simulink model "mvdc_KF_PointMassJoint"  (R2018b)
settings: configuration reference "Active" (kept outside this file)
undefined symbols (not defined in the file): P_VDC_EnableInputCrossCorrelation, P_VDC_InputCov, P_VDC_ManualInitializationStartPose, P_VDC_ManualInitializationStateEstimation, P_VDC_MeasCov, P_VDC_OutlierBounds, P_VDC_ResFilterSamples, P_VDC_resLim_psiLoc1_rad, P_VDC_resLim_psiLoc2_rad, P_VDC_resLim_vxVel1_mps, P_VDC_resLim_vxVel2_mps, P_VDC_resLim_vyVel1_mps, P_VDC_resLim_vyVel2_mps, P_VDC_resLim_xLoc1_m, P_VDC_resLim_xLoc2_m, P_VDC_resLim_yLoc1_m, P_VDC_resLim_yLoc2_m, P_VDC_YawAngleDepCovMode, res_dLoc1_m, res_dLoc2_m, res_dPsi1_radps, res_dPsi2_radps, res_psiLoc1_rad, res_psiLoc2_rad, res_sLoc1_m, res_sLoc2_m, res_vxVel1_mps, res_vxVel2_mps, res_vyVel1_mps, res_vyVel2_mps, res_xLoc1_m, res_xLoc2_m, res_yLoc1_m, res_yLoc2_m, tS
libraries: simulink x12
settings Model: DataDictionary=mvdc_KF_PointMassJoint.sldd  Creator=Madeline  LastModifiedBy=ge34qer

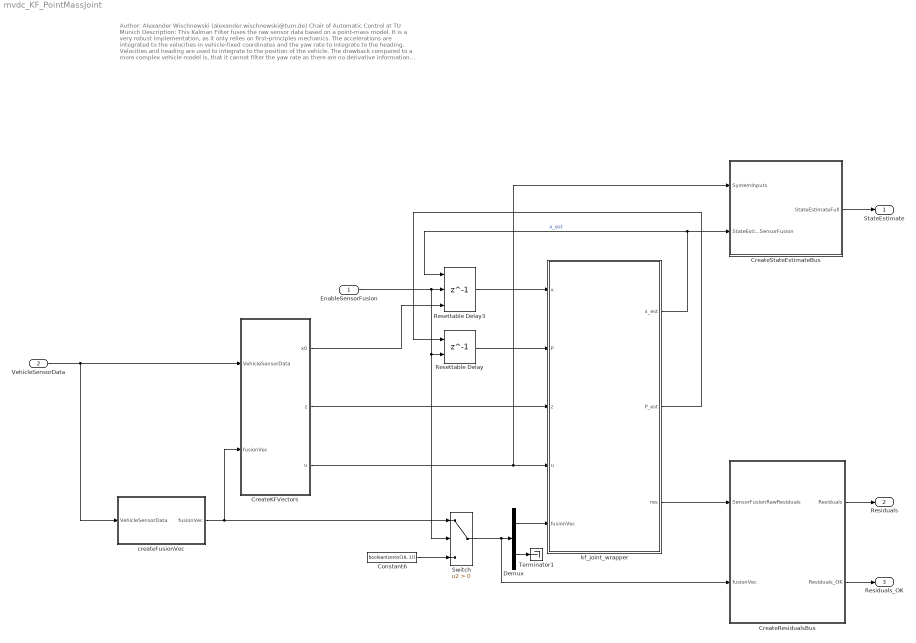
== system mvdc_KF_PointMassJoint ==
  note: Author: Alexander Wischnewski (alexander.wischnewski@tum.de)
      | Chair of Automatic Control at TU Munich
      |
      | Description: This Kalman Filter fuses the raw sensor data based on a point-mass model. It is a very robust implementation, as it only relies on first-principles mechanics. The accelerations are integrated to the velocities in vehicle-fixed coordinates and the yaw rate to integrate to the heading. Velocities and heading are used to integrate to the position of the vehicle. The drawback compared to a more complex vehicle model is, that it cannot filter the yaw rate as there are no derivative information about the yaw rate available. However, it is easy to tune and has comparable performance over the whole range of operating points.
      |
      | Inputs:
      | EnableSensorFusion Enable bit which activates the Kalman Filter
      | VehicleSensorData Raw sensor data
      |
      | Outputs:
      | StateEstimate Estimated state vector of the Kalman Filter
      | Residuals Pre-update measurement residuals of the Kalman Filter
      | Covariances Post-update Estimation Covariance Matrix of the Kalman Filter
  EnableSensorFusion : Inport  OutDataTypeStr=boolean
  VehicleSensorData : Inport  Port=2  OutDataTypeStr=Bus: VehicleSensorData
  Constant6 : Constant  Value=boolean(zeros(16, 1))
  CreateKFVectors : Subsystem
  CreateResidualsBus : Subsystem
  CreateStateEstimateBus : Subsystem
  Demux : Demux  Outputs=[10 6]
  Resettable Delay : Delay  DelayLength=1  InitialCondition=eye(5)*0.1  ExternalReset=Rising
      settings: InputPortMap=u0,r5
  Resettable Delay3 : Delay  DelayLength=1  InitialConditionSource=Input port  ExternalReset=Rising
      settings: InputPortMap=u0,r5,p4
  Switch : Switch  Criteria=u2 > Threshold
  Terminator1 : Terminator
  createFusionVec : Subsystem
  kf_joint_wrapper : MATLAB Function  TreatAsAtomicUnit=on
  "StateEstimate " : Outport  OutDataTypeStr=Bus: StateEstimation_state
  Residuals : Outport  Port=2  OutDataTypeStr=Bus: StateEstimation_residuals
  Residuals_OK : Outport  Port=3  OutDataTypeStr=boolean
  wires:
  kf_joint_wrapper/1(x_est) -> Resettable Delay3/1, CreateStateEstimateBus/2(StateEstimateSensorFusion)  "x_est"
  Resettable Delay3/1 -> kf_joint_wrapper/1(x)
  kf_joint_wrapper/2(P_est) -> Resettable Delay/1
  Resettable Delay/1 -> kf_joint_wrapper/2(P)
  CreateResidualsBus/1(Residuals) -> Residuals/1
  CreateKFVectors/1(x0) -> Resettable Delay3/3
  VehicleSensorData/1 -> createFusionVec/1(VehicleSensorData), CreateKFVectors/1(VehicleSensorData)
  CreateKFVectors/2(z) -> kf_joint_wrapper/3(z)
  CreateKFVectors/3(u) -> CreateStateEstimateBus/1(SystemInputs), kf_joint_wrapper/4(u)
  CreateStateEstimateBus/1(StateEstimateFull) -> "StateEstimate "/1
  kf_joint_wrapper/3(res) -> CreateResidualsBus/1(SensorFusionRawResiduals)
  Demux/2 -> Terminator1/1
  Demux/1 -> kf_joint_wrapper/5(fusionVec)
  Constant6/1 -> Switch/3
  EnableSensorFusion/1 -> Switch/2, Resettable Delay/2, Resettable Delay3/2
  createFusionVec/1(fusionVec) -> CreateKFVectors/2(fusionVec), Switch/1
  Switch/1 -> CreateResidualsBus/2(fusionVec), Demux/1
  CreateResidualsBus/2(Residuals_OK) -> Residuals_OK/1

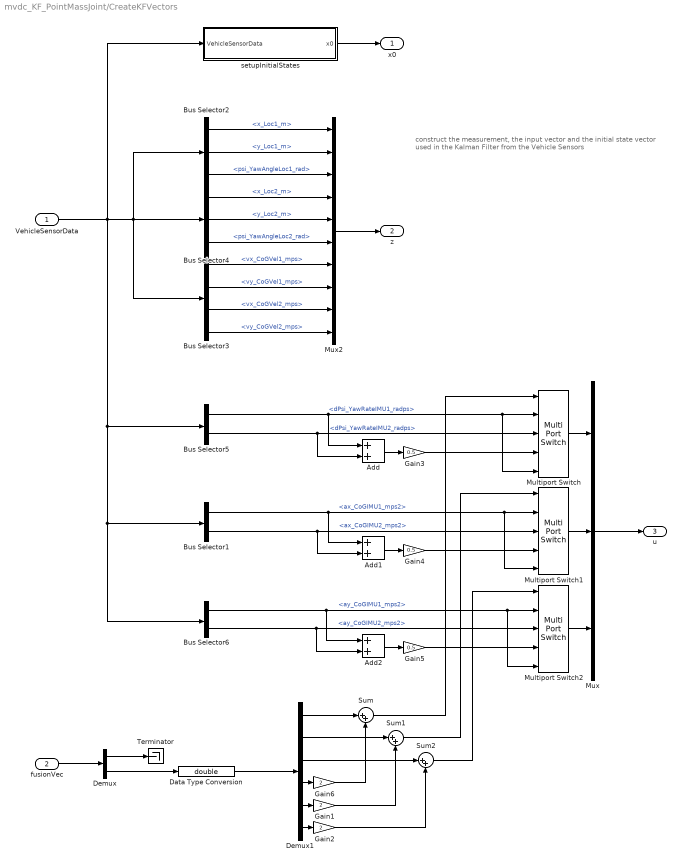
== system mvdc_KF_PointMassJoint/CreateKFVectors ==
  note: construct the measurement, the input vector and the initial state vector
      | used in the Kalman Filter from the Vehicle Sensors
  VehicleSensorData : Inport
  fusionVec : Inport  Port=2  OutDataTypeStr=boolean  PortDimensions=16
  Add : Sum
  Add1 : Sum
  Add2 : Sum
  Bus Selector1 : BusSelector  OutputSignals=ax_CoGIMU1_mps2,ax_CoGIMU2_mps2
  Bus Selector2 : BusSelector  OutputSignals=x_Loc1_m,y_Loc1_m,psi_YawAngleLoc1_rad
  Bus Selector3 : BusSelector  OutputSignals=vx_CoGVel1_mps,vy_CoGVel1_mps,vx_CoGVel2_mps,vy_CoGVel2_mps
  Bus Selector4 : BusSelector  OutputSignals=x_Loc2_m,y_Loc2_m,psi_YawAngleLoc2_rad
  Bus Selector5 : BusSelector  OutputSignals=dPsi_YawRateIMU1_radps,dPsi_YawRateIMU2_radps
  Bus Selector6 : BusSelector  OutputSignals=ay_CoGIMU1_mps2,ay_CoGIMU2_mps2
  Data Type Conversion : DataTypeConversion  OutDataTypeStr=double
  Demux : Demux  Outputs=[10 6]
  Demux1 : Demux  Outputs=6
  Gain1 : Gain  Gain=2
  Gain2 : Gain  Gain=2
  Gain3 : Gain  Gain=0.5
  Gain4 : Gain  Gain=0.5
  Gain5 : Gain  Gain=0.5
  Gain6 : Gain  Gain=2
  Multiport Switch : MultiPortSwitch  DataPortForDefault=Additional data port  DiagnosticForDefault=Warning
  Multiport Switch1 : MultiPortSwitch  DataPortForDefault=Additional data port  DiagnosticForDefault=Warning
  Multiport Switch2 : MultiPortSwitch  DataPortForDefault=Additional data port  DiagnosticForDefault=Warning
  Mux : Mux  Inputs=3
  Mux2 : Mux  Inputs=10
  Sum : Sum  Inputs=|++
  Sum1 : Sum  Inputs=|++
  Sum2 : Sum  Inputs=|++
  Terminator : Terminator
  setupInitialStates : Subsystem
  x0 : Outport
  z : Outport  Port=2
  u : Outport  Port=3
  wires:
  Mux2/1 -> z/1
  Bus Selector4/1 -> Mux2/4  "<x_Loc2_m>"
  Bus Selector4/2 -> Mux2/5  "<y_Loc2_m>"
  Bus Selector2/3 -> Mux2/3  "<psi_YawAngleLoc1_rad>"
  Bus Selector4/3 -> Mux2/6  "<psi_YawAngleLoc2_rad>"
  Bus Selector2/2 -> Mux2/2  "<y_Loc1_m>"
  Bus Selector2/1 -> Mux2/1  "<x_Loc1_m>"
  Bus Selector3/1 -> Mux2/7  "<vx_CoGVel1_mps>"
  Bus Selector3/2 -> Mux2/8  "<vy_CoGVel1_mps>"
  Bus Selector3/3 -> Mux2/9  "<vx_CoGVel2_mps>"
  Bus Selector3/4 -> Mux2/10  "<vy_CoGVel2_mps>"
  setupInitialStates/1(x0) -> x0/1
  Mux/1 -> u/1
  Demux/1 -> Terminator/1
  Demux/2 -> Data Type Conversion/1
  Demux1/6 -> Gain2/1
  Demux1/1 -> Sum/1
  Demux1/2 -> Sum1/1
  Demux1/3 -> Sum2/1
  Bus Selector5/1 -> Add/1, Multiport Switch/5, Multiport Switch/2  "<dPsi_YawRateIMU1_radps>"
  Bus Selector5/2 -> Add/2, Multiport Switch/3  "<dPsi_YawRateIMU2_radps>"
  Add/1 -> Gain3/1
  Sum/1 -> Multiport Switch/1
  Multiport Switch/1 -> Mux/1
  Multiport Switch1/1 -> Mux/2
  VehicleSensorData/1 -> setupInitialStates/1(VehicleSensorData), Bus Selector6/1, Bus Selector1/1, Bus Selector5/1, Bus Selector2/1, Bus Selector3/1, Bus Selector4/1
  Sum1/1 -> Multiport Switch1/1
  Bus Selector6/1 -> Add2/1, Multiport Switch2/5, Multiport Switch2/2  "<ay_CoGIMU1_mps2>"
  Add2/1 -> Gain5/1
  Gain5/1 -> Multiport Switch2/4
  Bus Selector6/2 -> Add2/2, Multiport Switch2/3  "<ay_CoGIMU2_mps2>"
  Multiport Switch2/1 -> Mux/3
  Sum2/1 -> Multiport Switch2/1
  Demux1/5 -> Gain1/1
  Demux1/4 -> Gain6/1
  Gain6/1 -> Sum/2
  Gain1/1 -> Sum1/2
  Gain2/1 -> Sum2/2
  Gain3/1 -> Multiport Switch/4
  Bus Selector1/2 -> Add1/2, Multiport Switch1/3  "<ax_CoGIMU2_mps2>"
  Add1/1 -> Gain4/1
  Bus Selector1/1 -> Add1/1, Multiport Switch1/5, Multiport Switch1/2  "<ax_CoGIMU1_mps2>"
  Gain4/1 -> Multiport Switch1/4
  Data Type Conversion/1 -> Demux1/1
  fusionVec/1 -> Demux/1

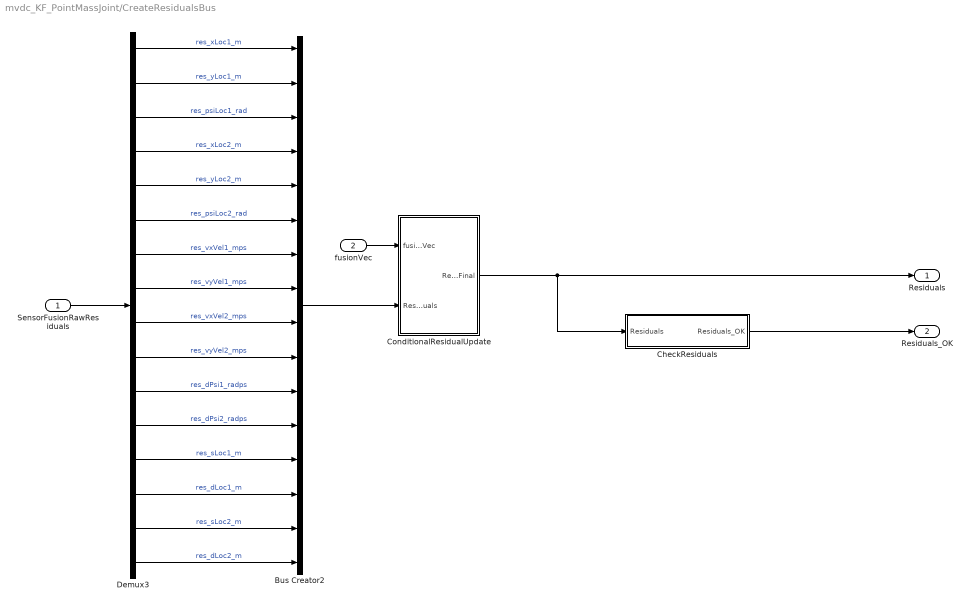
== system mvdc_KF_PointMassJoint/CreateResidualsBus ==
  SensorFusionRawResiduals : Inport
  fusionVec : Inport  Port=2
  Bus Creator2 : BusCreator  Inputs=16
  CheckResiduals : Subsystem
  ConditionalResidualUpdate : Subsystem
  Demux3 : Demux  Outputs=16
  Residuals : Outport
  Residuals_OK : Outport  Port=2  OutDataTypeStr=boolean
  wires:
  Demux3/3 -> Bus Creator2/3  "res_psiLoc1_rad"
  Demux3/1 -> Bus Creator2/1  "res_xLoc1_m"
  Demux3/2 -> Bus Creator2/2  "res_yLoc1_m"
  Demux3/13 -> Bus Creator2/13  "res_sLoc1_m"
  Demux3/14 -> Bus Creator2/14  "res_dLoc1_m"
  Demux3/15 -> Bus Creator2/15  "res_sLoc2_m"
  Demux3/16 -> Bus Creator2/16  "res_dLoc2_m"
  fusionVec/1 -> ConditionalResidualUpdate/1(fusionVec)
  SensorFusionRawResiduals/1 -> Demux3/1
  Bus Creator2/1 -> ConditionalResidualUpdate/2(Residuals)
  Demux3/4 -> Bus Creator2/4  "res_xLoc2_m"
  Demux3/5 -> Bus Creator2/5  "res_yLoc2_m"
  Demux3/6 -> Bus Creator2/6  "res_psiLoc2_rad"
  Demux3/7 -> Bus Creator2/7  "res_vxVel1_mps"
  Demux3/8 -> Bus Creator2/8  "res_vyVel1_mps"
  Demux3/11 -> Bus Creator2/11  "res_dPsi1_radps"
  Demux3/9 -> Bus Creator2/9  "res_vxVel2_mps"
  Demux3/10 -> Bus Creator2/10  "res_vyVel2_mps"
  Demux3/12 -> Bus Creator2/12  "res_dPsi2_radps"
  ConditionalResidualUpdate/1(ResidualsFinal) -> CheckResiduals/1(Residuals), Residuals/1
  CheckResiduals/1(Residuals_OK) -> Residuals_OK/1

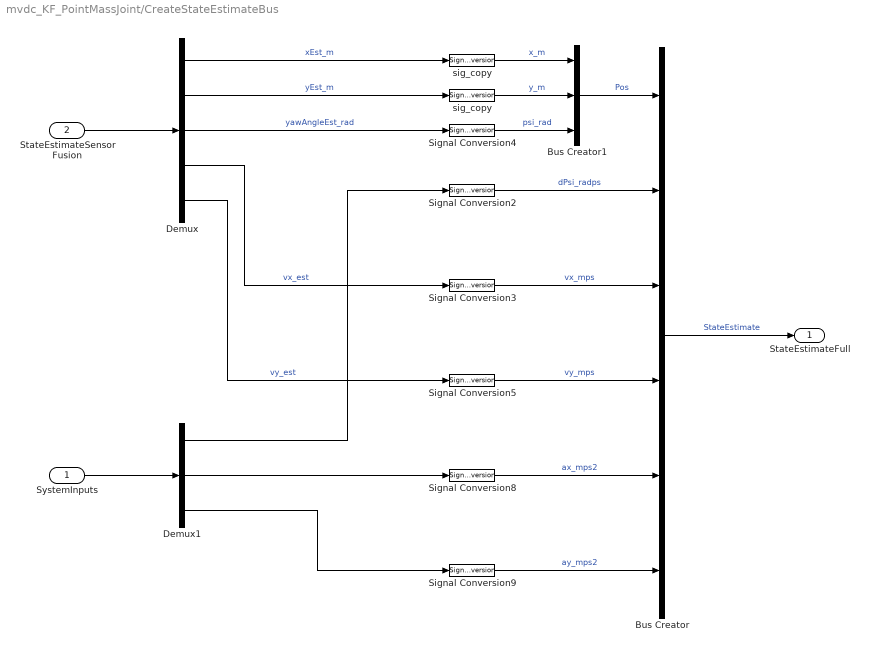
== system mvdc_KF_PointMassJoint/CreateStateEstimateBus ==
  SystemInputs : Inport
  StateEstimateSensorFusion : Inport  Port=2
  Bus Creator : BusCreator  Inputs=6
  Bus Creator1 : BusCreator  Inputs=3  OutDataTypeStr=Bus: CartPos
  Demux : Demux  Outputs=5
  Demux1 : Demux  Outputs=3
  Signal Conversion{2..5,8..9} (6 alike) : SignalConversion  OverrideOpt=off
  sig_copy : SignalConversion  OverrideOpt=off
  "sig_copy " : SignalConversion  OverrideOpt=off
  StateEstimateFull : Outport
  wires:
  StateEstimateSensorFusion/1 -> Demux/1
  Demux/1 -> "sig_copy "/1  "xEst_m"
  "sig_copy "/1 -> Bus Creator1/1  "x_m"
  Demux/3 -> Signal Conversion4/1  "yawAngleEst_rad"
  Demux/2 -> sig_copy/1  "yEst_m"
  Bus Creator/1 -> StateEstimateFull/1  "StateEstimate"
  Bus Creator1/1 -> Bus Creator/1  "Pos"
  Signal Conversion4/1 -> Bus Creator1/3  "psi_rad"
  Signal Conversion3/1 -> Bus Creator/3  "vx_mps"
  Signal Conversion2/1 -> Bus Creator/2  "dPsi_radps"
  Signal Conversion8/1 -> Bus Creator/5  "ax_mps2"
  Signal Conversion9/1 -> Bus Creator/6  "ay_mps2"
  Signal Conversion5/1 -> Bus Creator/4  "vy_mps"
  sig_copy/1 -> Bus Creator1/2  "y_m"
  Demux/5 -> Signal Conversion5/1  "vy_est"
  Demux/4 -> Signal Conversion3/1  "vx_est"
  SystemInputs/1 -> Demux1/1
  Demux1/1 -> Signal Conversion2/1
  Demux1/2 -> Signal Conversion8/1
  Demux1/3 -> Signal Conversion9/1

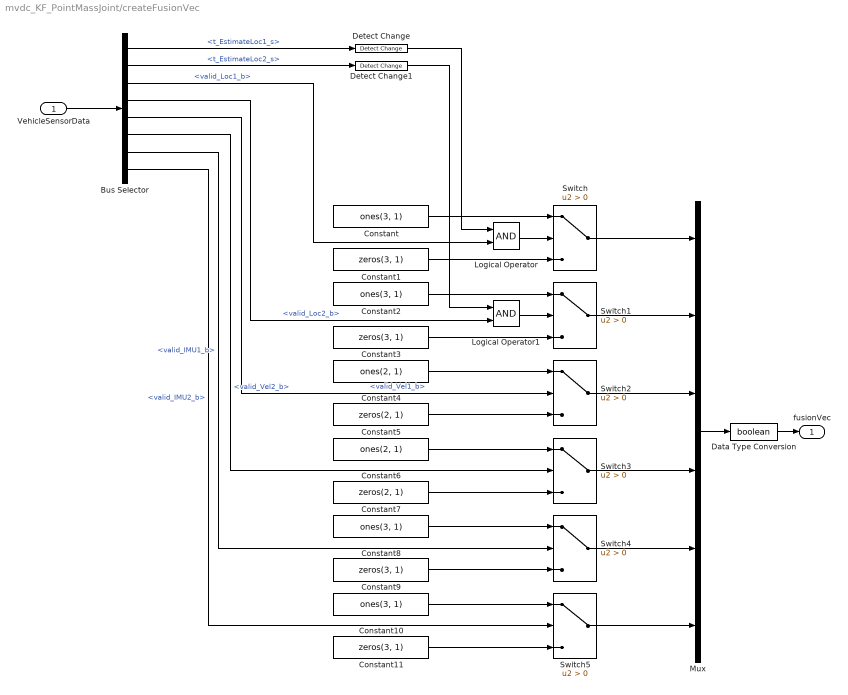
== system mvdc_KF_PointMassJoint/createFusionVec ==
  VehicleSensorData : Inport
  Bus Selector : BusSelector  OutputSignals=t_EstimateLoc1_s,t_EstimateLoc2_s,valid_Loc1_b,valid_Loc2_b,valid_Vel1_b,valid_Vel2_b,valid_IMU1_b,valid_IMU2_b
  Constant{,2,8,10} (4 alike) : Constant  Value=ones(3, 1)
  Constant{1,3,9,11} (4 alike) : Constant  Value=zeros(3, 1)
  Constant4 : Constant  Value=ones(2, 1)
  Constant5 : Constant  Value=zeros(2, 1)
  Constant6 : Constant  Value=ones(2, 1)
  Constant7 : Constant  Value=zeros(2, 1)
  Data Type Conversion : DataTypeConversion  OutDataTypeStr=boolean
  Detect Change : simulink/Logic and Bit Operations/Detect Change  vinit=0  OutDataTypeStr=boolean
  Detect Change1 : simulink/Logic and Bit Operations/Detect Change  vinit=0  OutDataTypeStr=boolean
  Logical Operator : Logic  AllPortsSameDT=off  OutDataTypeStr=boolean
  Logical Operator1 : Logic  AllPortsSameDT=off  OutDataTypeStr=boolean
  Mux : Mux  Inputs=6
  Switch{,1..5} (6 alike) : Switch  Criteria=u2 > Threshold
  fusionVec : Outport
  wires:
  Switch5/1 -> Mux/6
  Constant7/1 -> Switch3/3
  Switch2/1 -> Mux/3
  Constant8/1 -> Switch4/1
  Constant6/1 -> Switch3/1
  Constant1/1 -> Switch/3
  Constant2/1 -> Switch1/1
  Constant11/1 -> Switch5/3
  Switch3/1 -> Mux/4
  Switch4/1 -> Mux/5
  Constant9/1 -> Switch4/3
  Constant5/1 -> Switch2/3
  Constant/1 -> Switch/1
  Constant10/1 -> Switch5/1
  Switch/1 -> Mux/1
  Constant4/1 -> Switch2/1
  Switch1/1 -> Mux/2
  Constant3/1 -> Switch1/3
  Data Type Conversion/1 -> fusionVec/1
  Mux/1 -> Data Type Conversion/1
  Logical Operator/1 -> Switch/2
  Logical Operator1/1 -> Switch1/2
  VehicleSensorData/1 -> Bus Selector/1
  Bus Selector/1 -> Detect Change/1  "<t_EstimateLoc1_s>"
  Bus Selector/2 -> Detect Change1/1  "<t_EstimateLoc2_s>"
  Detect Change/1 -> Logical Operator/1
  Detect Change1/1 -> Logical Operator1/1
  Bus Selector/3 -> Logical Operator/2  "<valid_Loc1_b>"
  Bus Selector/4 -> Logical Operator1/2  "<valid_Loc2_b>"
  Bus Selector/5 -> Switch2/2  "<valid_Vel1_b>"
  Bus Selector/6 -> Switch3/2  "<valid_Vel2_b>"
  Bus Selector/7 -> Switch4/2  "<valid_IMU1_b>"
  Bus Selector/8 -> Switch5/2  "<valid_IMU2_b>"

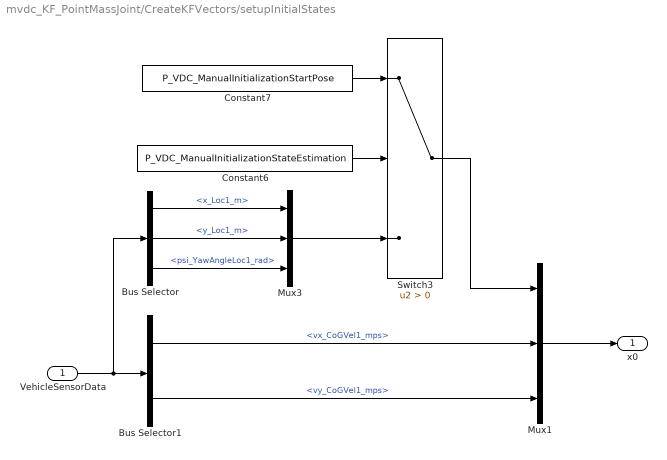
== system mvdc_KF_PointMassJoint/CreateKFVectors/setupInitialStates ==
  VehicleSensorData : Inport
  Bus Selector : BusSelector  OutputSignals=x_Loc1_m,y_Loc1_m,psi_YawAngleLoc1_rad
  Bus Selector1 : BusSelector  OutputSignals=vx_CoGVel1_mps,vy_CoGVel1_mps
  Constant6 : Constant  Value=P_VDC_ManualInitializationStateEstimation
  Constant7 : Constant  Value=P_VDC_ManualInitializationStartPose
  Mux1 : Mux  Inputs=3
  Mux3 : Mux  Inputs=3
  Switch3 : Switch  Criteria=u2 > Threshold
  x0 : Outport
  wires:
  Bus Selector/1 -> Mux3/1  "<x_Loc1_m>"
  Bus Selector1/1 -> Mux1/2  "<vx_CoGVel1_mps>"
  VehicleSensorData/1 -> Bus Selector/1, Bus Selector1/1
  Constant6/1 -> Switch3/2
  Mux3/1 -> Switch3/3
  Bus Selector/2 -> Mux3/2  "<y_Loc1_m>"
  Bus Selector1/2 -> Mux1/3  "<vy_CoGVel1_mps>"
  Switch3/1 -> Mux1/1
  Constant7/1 -> Switch3/1
  Bus Selector/3 -> Mux3/3  "<psi_YawAngleLoc1_rad>"
  Mux1/1 -> x0/1

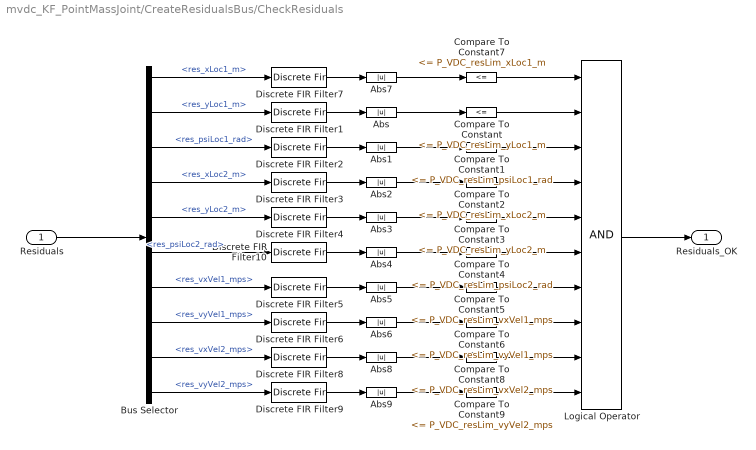
== system mvdc_KF_PointMassJoint/CreateResidualsBus/CheckResiduals ==
  Residuals : Inport
  Abs{,1..9} (10 alike) : Abs
  Bus Selector : BusSelector  OutputSignals=res_xLoc1_m,res_yLoc1_m,res_psiLoc1_rad,res_xLoc2_m,res_yLoc2_m,res_psiLoc2_rad,res_vxVel1_mps,res_vyVel1_mps,res_vxVel2_mps,res_vyVel2_mps
  Compare To Constant : simulink/Logic and Bit Operations/Compare To Constant  relop=<=  const=P_VDC_resLim_yLoc1_m  OutDataTypeStr=boolean
  Compare To Constant1 : simulink/Logic and Bit Operations/Compare To Constant  relop=<=  const=P_VDC_resLim_psiLoc1_rad  OutDataTypeStr=boolean
  Compare To Constant2 : simulink/Logic and Bit Operations/Compare To Constant  relop=<=  const=P_VDC_resLim_xLoc2_m  OutDataTypeStr=boolean
  Compare To Constant3 : simulink/Logic and Bit Operations/Compare To Constant  relop=<=  const=P_VDC_resLim_yLoc2_m  OutDataTypeStr=boolean
  Compare To Constant4 : simulink/Logic and Bit Operations/Compare To Constant  relop=<=  const=P_VDC_resLim_psiLoc2_rad  OutDataTypeStr=boolean
  Compare To Constant5 : simulink/Logic and Bit Operations/Compare To Constant  relop=<=  const=P_VDC_resLim_vxVel1_mps  OutDataTypeStr=boolean
  Compare To Constant6 : simulink/Logic and Bit Operations/Compare To Constant  relop=<=  const=P_VDC_resLim_vyVel1_mps  OutDataTypeStr=boolean
  Compare To Constant7 : simulink/Logic and Bit Operations/Compare To Constant  relop=<=  const=P_VDC_resLim_xLoc1_m  OutDataTypeStr=boolean
  Compare To Constant8 : simulink/Logic and Bit Operations/Compare To Constant  relop=<=  const=P_VDC_resLim_vxVel2_mps  OutDataTypeStr=boolean
  Compare To Constant9 : simulink/Logic and Bit Operations/Compare To Constant  relop=<=  const=P_VDC_resLim_vyVel2_mps  OutDataTypeStr=boolean
  Discrete FIR Filter{1..10} (10 alike) : DiscreteFir  Coefficients=ones(1, P_VDC_ResFilterSamples)/P_VDC_ResFilterSamples
  Logical Operator : Logic  Inputs=10  AllPortsSameDT=off  OutDataTypeStr=boolean
  Residuals_OK : Outport
  wires:
  Bus Selector/10 -> Discrete FIR Filter9/1  "<res_vyVel2_mps>"
  Abs7/1 -> Compare To Constant7/1
  Abs9/1 -> Compare To Constant9/1
  Abs6/1 -> Compare To Constant6/1
  Discrete FIR Filter3/1 -> Abs2/1
  Bus Selector/2 -> Discrete FIR Filter1/1  "<res_yLoc1_m>"
  Compare To Constant/1 -> Logical Operator/2
  Compare To Constant8/1 -> Logical Operator/9
  Bus Selector/1 -> Discrete FIR Filter7/1  "<res_xLoc1_m>"
  Bus Selector/7 -> Discrete FIR Filter5/1  "<res_vxVel1_mps>"
  Compare To Constant9/1 -> Logical Operator/10
  Bus Selector/3 -> Discrete FIR Filter2/1  "<res_psiLoc1_rad>"
  Compare To Constant5/1 -> Logical Operator/7
  Bus Selector/8 -> Discrete FIR Filter6/1  "<res_vyVel1_mps>"
  Abs8/1 -> Compare To Constant8/1
  Discrete FIR Filter1/1 -> Abs/1
  Bus Selector/9 -> Discrete FIR Filter8/1  "<res_vxVel2_mps>"
  Discrete FIR Filter9/1 -> Abs9/1
  Bus Selector/6 -> Discrete FIR Filter10/1  "<res_psiLoc2_rad>"
  Abs/1 -> Compare To Constant/1
  Residuals/1 -> Bus Selector/1
  Discrete FIR Filter7/1 -> Abs7/1
  Abs1/1 -> Compare To Constant1/1
  Abs2/1 -> Compare To Constant2/1
  Discrete FIR Filter10/1 -> Abs4/1
  Compare To Constant2/1 -> Logical Operator/4
  Bus Selector/4 -> Discrete FIR Filter3/1  "<res_xLoc2_m>"
  Abs5/1 -> Compare To Constant5/1
  Compare To Constant6/1 -> Logical Operator/8
  Discrete FIR Filter8/1 -> Abs8/1
  Discrete FIR Filter5/1 -> Abs5/1
  Abs3/1 -> Compare To Constant3/1
  Discrete FIR Filter6/1 -> Abs6/1
  Compare To Constant7/1 -> Logical Operator/1
  Bus Selector/5 -> Discrete FIR Filter4/1  "<res_yLoc2_m>"
  Discrete FIR Filter4/1 -> Abs3/1
  Abs4/1 -> Compare To Constant4/1
  Compare To Constant3/1 -> Logical Operator/5
  Compare To Constant1/1 -> Logical Operator/3
  Discrete FIR Filter2/1 -> Abs1/1
  Compare To Constant4/1 -> Logical Operator/6
  Logical Operator/1 -> Residuals_OK/1

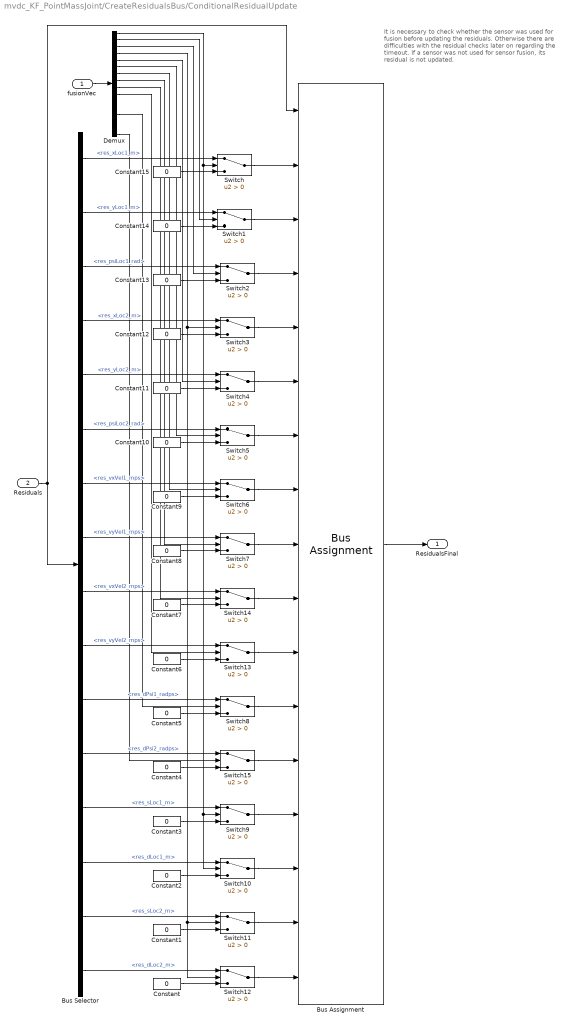
== system mvdc_KF_PointMassJoint/CreateResidualsBus/ConditionalResidualUpdate ==
  note: It is necessary to check
      | whether the sensor was used for fusion
      | before updating the residuals. Otherwise
      | there are difficulties with the residual checks
      | later on regarding the timeout. If a sensor was
      | not used for sensor fusion, its residual is not updated.
  fusionVec : Inport
  Residuals : Inport  Port=2
  Bus Assignment : BusAssignment  AssignedSignals=res_xLoc1_m,res_yLoc1_m,res_psiLoc1_rad,res_xLoc2_m,res_yLoc2_m,res_psiLoc2_rad,res_vxVel1_mps,res_vyVel1_mps,res_vxVel2_mps,res_vyVel2_mps,res_dPsi1_radps,res_dPsi2_radps,res_sLoc1_m,res_dLoc1_m,res_sLoc2_m,res_dLoc2_m
  Bus Selector : BusSelector  OutputSignals=res_xLoc1_m,res_yLoc1_m,res_psiLoc1_rad,res_xLoc2_m,res_yLoc2_m,res_psiLoc2_rad,res_vxVel1_mps,res_vyVel1_mps,res_vxVel2_mps,res_vyVel2_mps,res_dPsi1_radps,res_dPsi2_radps,res_sLoc1_m,res_dLoc1_m,res_sLoc2_m,res_dLoc2_m
  Constant{,1..15} (16 alike) : Constant  Value=0
  Demux : Demux  Outputs=16
  Switch{,1..15} (16 alike) : Switch  Criteria=u2 > Threshold
  ResidualsFinal : Outport
  wires:
  Demux/5 -> Switch4/2
  Switch8/1 -> Bus Assignment/12
  Bus Selector/6 -> Switch5/1  "<res_psiLoc2_rad>"
  Switch6/1 -> Bus Assignment/8
  Demux/7 -> Switch6/2
  Switch7/1 -> Bus Assignment/9
  Switch2/1 -> Bus Assignment/4
  Switch4/1 -> Bus Assignment/6
  Switch/1 -> Bus Assignment/2
  Bus Assignment/1 -> ResidualsFinal/1
  Demux/3 -> Switch2/2
  Residuals/1 -> Bus Assignment/1, Bus Selector/1
  Bus Selector/1 -> Switch/1  "<res_xLoc1_m>"
  Demux/8 -> Switch7/2
  Switch5/1 -> Bus Assignment/7
  Demux/2 -> Switch1/2
  Demux/6 -> Switch5/2
  Demux/4 -> Switch12/2, Switch11/2, Switch3/2
  Bus Selector/8 -> Switch7/1  "<res_vyVel1_mps>"
  Bus Selector/7 -> Switch6/1  "<res_vxVel1_mps>"
  Bus Selector/2 -> Switch1/1  "<res_yLoc1_m>"
  Switch1/1 -> Bus Assignment/3
  fusionVec/1 -> Demux/1
  Bus Selector/11 -> Switch8/1  "<res_dPsi1_radps>"
  Switch12/1 -> Bus Assignment/17
  Switch10/1 -> Bus Assignment/15
  Switch11/1 -> Bus Assignment/16
  Switch9/1 -> Bus Assignment/14
  Bus Selector/13 -> Switch9/1  "<res_sLoc1_m>"
  Bus Selector/16 -> Switch12/1  "<res_dLoc2_m>"
  Bus Selector/15 -> Switch11/1  "<res_sLoc2_m>"
  Bus Selector/14 -> Switch10/1  "<res_dLoc1_m>"
  Demux/1 -> Switch/2, Switch10/2, Switch9/2
  Bus Selector/3 -> Switch2/1  "<res_psiLoc1_rad>"
  Bus Selector/4 -> Switch3/1  "<res_xLoc2_m>"
  Bus Selector/5 -> Switch4/1  "<res_yLoc2_m>"
  Switch3/1 -> Bus Assignment/5
  Switch13/1 -> Bus Assignment/11
  Bus Selector/10 -> Switch13/1  "<res_vyVel2_mps>"
  Switch14/1 -> Bus Assignment/10
  Bus Selector/9 -> Switch14/1  "<res_vxVel2_mps>"
  Demux/9 -> Switch14/2
  Demux/10 -> Switch13/2
  Bus Selector/12 -> Switch15/1  "<res_dPsi2_radps>"
  Demux/13 -> Switch8/2
  Switch15/1 -> Bus Assignment/13
  Demux/16 -> Switch15/2
  Constant/1 -> Switch12/3
  Constant1/1 -> Switch11/3
  Constant2/1 -> Switch10/3
  Constant3/1 -> Switch9/3
  Constant4/1 -> Switch15/3
  Constant5/1 -> Switch8/3
  Constant6/1 -> Switch13/3
  Constant7/1 -> Switch14/3
  Constant8/1 -> Switch7/3
  Constant9/1 -> Switch6/3
  Constant10/1 -> Switch5/3
  Constant11/1 -> Switch4/3
  Constant12/1 -> Switch3/3
  Constant13/1 -> Switch2/3
  Constant14/1 -> Switch1/3
  Constant15/1 -> Switch/3

== matlab function mvdc_KF_PointMassJoint/kf_joint_wrapper ==
  data: x input; P input; z input; u input; fusionVec input boolean size=10; tS parameter; P_VDC_InputCov parameter; P_VDC_OutlierBounds parameter; P_VDC_YawAngleDepCovMode parameter; P_VDC_EnableInputCrossCorrelation parameter; x_est output; P_est output; res output size=16; P_VDC_MeasCov parameter size=10
function [x_est, P_est, res] = kf_joint_wrapper(x, P, z, u, fusionVec, tS, P_VDC_InputCov, P_VDC_OutlierBounds, P_VDC_YawAngleDepCovMode, P_VDC_EnableInputCrossCorrelation, P_VDC_MeasCov)

[x_est, P_est, res]= kf_joint(x, P, z, u, fusionVec, tS, P_VDC_InputCov, P_VDC_OutlierBounds, P_VDC_YawAngleDepCovMode, P_VDC_EnableInputCrossCorrelation, P_VDC_MeasCov);

end
